simulink model "BikeModelTranslationToHitch"  (Simulink 7.7)
settings: Solver=ode1  StartTime=0.0  StopTime=30  FixedStep=1e-3  RelTol=1e-3
undefined symbols (not defined in the file): Df, L1, L12, v
settings Model: Creator=Raul  LastModifiedBy=Raul

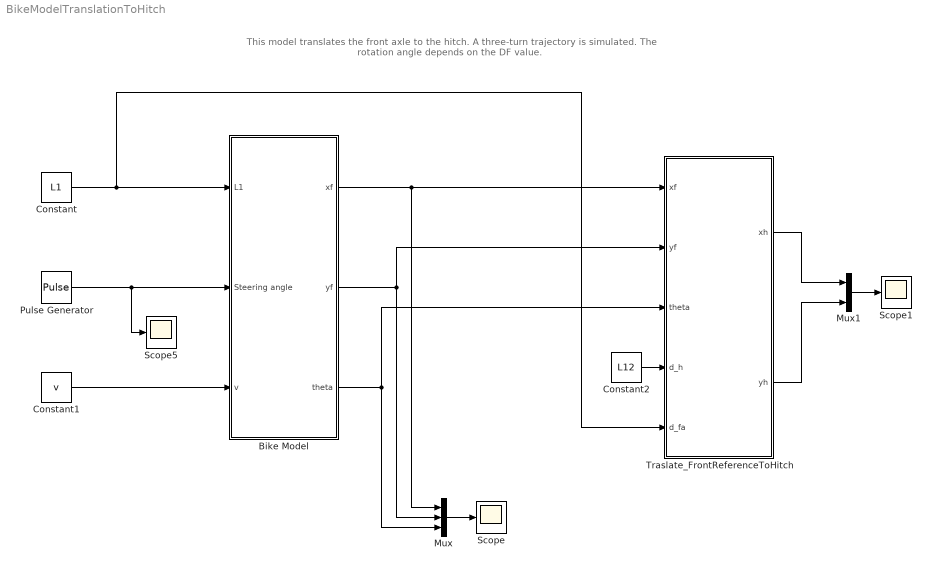
== system BikeModelTranslationToHitch ==
  note: This model translates the front axle to the hitch. A three-turn trajectory is simulated. The rotation angle depends on the DF value.
  "Bike Model " : Subsystem
  Constant : Constant  Value=L1
  Constant1 : Constant  Value=v
  Constant2 : Constant  Value=L12
  Mux : Mux  Inputs=3
  Mux1 : Mux  Inputs=2
  Pulse Generator : DiscretePulseGenerator  PulseType=Time based  Amplitude=Df  Period=10  PulseWidth=60  PhaseDelay=2
  Scope : Scope
  Scope1 : Scope
  Scope5 : Scope
      settings: SaveName=ScopeData5
  Traslate_FrontReferenceToHitch : Stateflow chart  TreatAsAtomicUnit=on
  wires:
  Constant/1 -> "Bike Model "/1(L1), Traslate_FrontReferenceToHitch/5(d_fa)
  Constant1/1 -> "Bike Model "/3(v)
  Mux/1 -> Scope/1
  "Bike Model "/1(xf) -> Mux/1, Traslate_FrontReferenceToHitch/1(xf)
  "Bike Model "/2(yf) -> Mux/2, Traslate_FrontReferenceToHitch/2(yf)
  "Bike Model "/3(theta) -> Mux/3, Traslate_FrontReferenceToHitch/3(theta)
  Constant2/1 -> Traslate_FrontReferenceToHitch/4(d_h)
  Mux1/1 -> Scope1/1
  Traslate_FrontReferenceToHitch/1(xh) -> Mux1/1
  Traslate_FrontReferenceToHitch/2(yh) -> Mux1/2
  Pulse Generator/1 -> "Bike Model "/2(Steering angle), Scope5/1

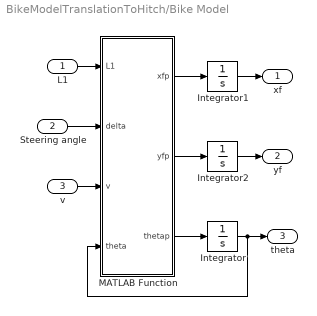
== system BikeModelTranslationToHitch/Bike Model  ==
  L1 : Inport
  Steering angle : Inport  Port=2
  v : Inport  Port=3
  Integrator : Integrator
  Integrator1 : Integrator
  Integrator2 : Integrator
  MATLAB Function : Stateflow chart  TreatAsAtomicUnit=on
  xf : Outport
  yf : Outport  Port=2
  theta : Outport  Port=3
  wires:
  Integrator/1 -> MATLAB Function/4(theta), theta/1
  MATLAB Function/1(xfp) -> Integrator1/1
  MATLAB Function/2(yfp) -> Integrator2/1
  MATLAB Function/3(thetap) -> Integrator/1
  Steering angle/1 -> MATLAB Function/2(delta)
  L1/1 -> MATLAB Function/1(L1)
  Integrator1/1 -> xf/1
  Integrator2/1 -> yf/1
  v/1 -> MATLAB Function/3(v)

== matlab function Traslate_FrontReferenceToHitch ==
  data: xf input double; xh output double; yf input double; theta input double; d_h input double; yh output double; d_fa input double
function [xh,yh]= fcn(xf,yf,theta,d_h,d_fa)
%#codegen
xh=xf+(d_h+d_fa)*-cos(theta);
yh=yf+(d_h+d_fa)*-sin(theta);

== matlab function Bike Model /MATLAB Function ==
  data: L1 input double; xfp output double; delta input double; v input double; theta input double; yfp output double; thetap output double
function [xfp,yfp,thetap] = fcn(L1,delta,v,theta)
%#codegen
thetap=(v*sin(delta))/L1;
xfp=v*cos(theta+delta);
yfp=v*sin(theta+delta);
